simulink model "Lecture16_massSpringDamper"  (R2017b)
settings: Solver=VariableStepAuto  StartTime=0.0  StopTime=10.0  RelTol=1e-3
undefined symbols (not defined in the file): k, k2, x0
settings Model: Creator=jtb32  LastModifiedBy=jtb32

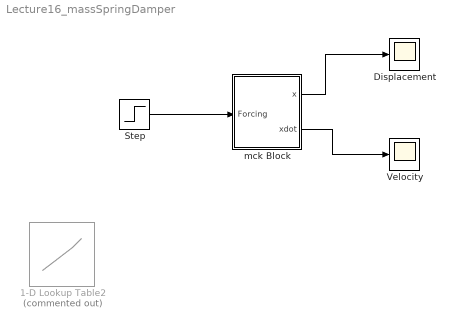
== system Lecture16_massSpringDamper ==
  1-D Lookup Table2 : Lookup_n-D  Commented=on  NumberOfTableDimensions=1  BreakpointsForDimension1=[-2*x0,-x0,x0,2*x0]  Table=[-(k+k2)*x0,-k*x0,k*x0,(k+k2)*x0]  InternalRulePriority=Speed  RndMeth=Simplest  InputSameDT=on
  Displacement : Scope
  Step : Step  After=1000  SampleTime=0
  Velocity : Scope
  "mck Block " : Subsystem  mask{m=250, c=1000, k=10000}
      mask prompts: m "Mass"; c "Damping Rate"; k "Spring Stiffness"
  wires:
  Step/1 -> "mck Block "/1(Forcing)
  "mck Block "/1(x) -> Displacement/1
  "mck Block "/2(xdot) -> Velocity/1

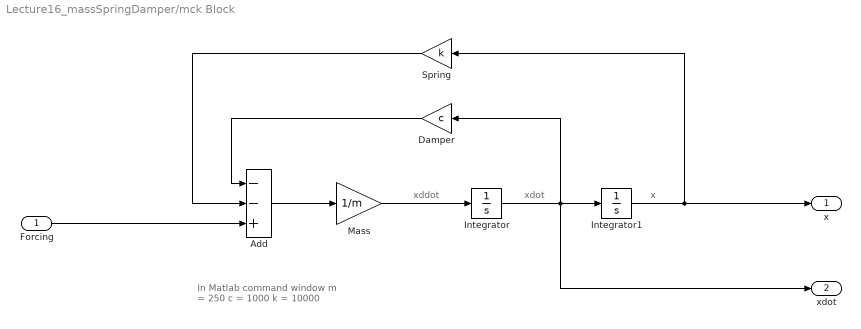
== system Lecture16_massSpringDamper/mck Block  ==
  note: In Matlab command window
      | m = 250
      | c = 1000
      | k = 10000
  note: x
  note: xddot
  note: xdot
  Forcing : Inport
  Add : Sum  Inputs=--+
  "Damper " : Gain  Gain=c
  Integrator : Integrator
  Integrator1 : Integrator
  Mass : Gain  Gain=1/m
  Spring : Gain  Gain=k
  x : Outport
  xdot : Outport  Port=2
  wires:
  Mass/1 -> Integrator/1
  Integrator1/1 -> x/1, Spring/1
  Integrator/1 -> xdot/1, "Damper "/1, Integrator1/1
  Add/1 -> Mass/1
  "Damper "/1 -> Add/1
  Spring/1 -> Add/2
  Forcing/1 -> Add/3
